simulink library "GenTil_Lib"  (R2023a)
settings: Solver=VariableStepAuto  StartTime=0.0  StopTime=10.0  RelTol=1e-3
values from neighbouring files (symbols this model uses):
  D = [0	0	0	0	0	0	0	0	0	0	0 ... (first row only)    [GenTil.m]
undefined symbols (not defined in the file or in its folder): aircraft, p, phi, psi, q, r, theta, v, w, x, y, z
libraries: simulink_extras x35, simulink x5, matrix_library x4, aerolibatmos2 x1
(part 2 of 2)

== system GenTil_Lib/GenTil/GenTil_Dynamics/Equations_of_Motion_6DoF/Dynamics/Moments/  ==
  note: In mathematics, a skew symmetric matrix is defined as the square matrix that is equal to the negative of its transpose matrix.
      | For any square matrix, A, the transpose matrix is given as A T . A skew-symmetric or antisymmetric matrix A can therefore be represented as, A = -A T .
  X : Inport
  Constant : Constant  Value=0
  Constant1 : Constant  Value=0
  Constant2 : Constant  Value=0
  Demux : Demux  Outputs=3
  From : From
  From1 : From
  Gain3 : Gain  Gain=-1
  Gain4 : Gain  Gain=-1
  Gain5 : Gain  Gain=-1
  Goto : Goto
  Matrix Concatenate3 : Concatenate  NumInputs=3  Mode=Multidimensional array  ConcatenateDimension=2
  Matrix Concatenate4 : Concatenate  NumInputs=3  Mode=Multidimensional array  ConcatenateDimension=2
  Matrix Concatenate5 : Concatenate  NumInputs=3  Mode=Multidimensional array  ConcatenateDimension=2
  Matrix Concatenate6 : Concatenate  NumInputs=3  Mode=Multidimensional array
  skew(x) : Outport
  wires:
  Constant2/1 -> Matrix Concatenate5/3
  Constant1/1 -> Matrix Concatenate4/2
  Constant/1 -> Matrix Concatenate3/1
  Demux/1 -> Goto/1
  Demux/2 -> [B]
  X/1 -> Demux/1
  [B] -> Gain4/1
  From1/1 -> Matrix Concatenate5/2
  Matrix Concatenate3/1 -> Matrix Concatenate6/1
  Demux/3 -> [C]
  [B] -> Matrix Concatenate3/3
  Matrix Concatenate5/1 -> Matrix Concatenate6/3
  Matrix Concatenate6/1 -> skew(x)/1  "skew(x)"
  Gain4/1 -> Matrix Concatenate5/1
  [C] -> Gain5/1
  [C] -> Matrix Concatenate4/1
  Gain3/1 -> Matrix Concatenate4/3
  From/1 -> Gain3/1
  Matrix Concatenate4/1 -> Matrix Concatenate6/2
  Gain5/1 -> Matrix Concatenate3/2

== system GenTil_Lib/GenTil/GenTil_Dynamics/Equations_of_Motion_6DoF/Dynamics/Moments/   ==
  note: In mathematics, a skew symmetric matrix is defined as the square matrix that is equal to the negative of its transpose matrix.
      | For any square matrix, A, the transpose matrix is given as A T . A skew-symmetric or antisymmetric matrix A can therefore be represented as, A = -A T .
  X : Inport
  Constant : Constant  Value=0
  Constant1 : Constant  Value=0
  Constant2 : Constant  Value=0
  Demux : Demux  Outputs=3
  From : From
  From1 : From
  Gain3 : Gain  Gain=-1
  Gain4 : Gain  Gain=-1
  Gain5 : Gain  Gain=-1
  Goto : Goto
  Matrix Concatenate3 : Concatenate  NumInputs=3  Mode=Multidimensional array  ConcatenateDimension=2
  Matrix Concatenate4 : Concatenate  NumInputs=3  Mode=Multidimensional array  ConcatenateDimension=2
  Matrix Concatenate5 : Concatenate  NumInputs=3  Mode=Multidimensional array  ConcatenateDimension=2
  Matrix Concatenate6 : Concatenate  NumInputs=3  Mode=Multidimensional array
  skew(x) : Outport
  wires:
  Constant2/1 -> Matrix Concatenate5/3
  Constant1/1 -> Matrix Concatenate4/2
  Constant/1 -> Matrix Concatenate3/1
  Demux/1 -> Goto/1
  Demux/2 -> [B]
  X/1 -> Demux/1
  [B] -> Gain4/1
  From1/1 -> Matrix Concatenate5/2
  Matrix Concatenate3/1 -> Matrix Concatenate6/1
  Demux/3 -> [C]
  [B] -> Matrix Concatenate3/3
  Matrix Concatenate5/1 -> Matrix Concatenate6/3
  Matrix Concatenate6/1 -> skew(x)/1  "skew(x)"
  Gain4/1 -> Matrix Concatenate5/1
  [C] -> Gain5/1
  [C] -> Matrix Concatenate4/1
  Gain3/1 -> Matrix Concatenate4/3
  From/1 -> Gain3/1
  Matrix Concatenate4/1 -> Matrix Concatenate6/2
  Gain5/1 -> Matrix Concatenate3/2

== system GenTil_Lib/GenTil/GenTil_Dynamics/Equations_of_Motion_6DoF/Dynamics/Moments/      ==
  attitude_angles_rad : Inport
  Product1 : Product  Inputs=3  Multiplication=Matrix(*)
  Subsystem : Subsystem
  C_bv : Outport  PortDimensions=[3,3]
  wires:
  attitude_angles_rad/1 -> Subsystem/1(attitude_angles_rad)
  Product1/1 -> C_bv/1
  Subsystem/3(C_psi) -> Product1/3
  Subsystem/1(C_phi) -> Product1/1
  Subsystem/2(C_theta) -> Product1/2

== system GenTil_Lib/GenTil/GenTil_Dynamics/Equations_of_Motion_6DoF/Dynamics/Moments/ 1 ==
  note: In mathematics, a skew symmetric matrix is defined as the square matrix that is equal to the negative of its transpose matrix.
      | For any square matrix, A, the transpose matrix is given as A T . A skew-symmetric or antisymmetric matrix A can therefore be represented as, A = -A T .
  X : Inport
  Constant : Constant  Value=0
  Constant1 : Constant  Value=0
  Constant2 : Constant  Value=0
  Demux : Demux  Outputs=3
  From : From
  From1 : From
  Gain3 : Gain  Gain=-1
  Gain4 : Gain  Gain=-1
  Gain5 : Gain  Gain=-1
  Goto : Goto
  Matrix Concatenate3 : Concatenate  NumInputs=3  Mode=Multidimensional array  ConcatenateDimension=2
  Matrix Concatenate4 : Concatenate  NumInputs=3  Mode=Multidimensional array  ConcatenateDimension=2
  Matrix Concatenate5 : Concatenate  NumInputs=3  Mode=Multidimensional array  ConcatenateDimension=2
  Matrix Concatenate6 : Concatenate  NumInputs=3  Mode=Multidimensional array
  skew(x) : Outport
  wires:
  Gain5/1 -> Matrix Concatenate3/2
  Matrix Concatenate4/1 -> Matrix Concatenate6/2
  From/1 -> Gain3/1
  Gain3/1 -> Matrix Concatenate4/3
  [C] -> Matrix Concatenate4/1
  [C] -> Gain5/1
  Gain4/1 -> Matrix Concatenate5/1
  Matrix Concatenate6/1 -> skew(x)/1  "skew(x)"
  Matrix Concatenate5/1 -> Matrix Concatenate6/3
  [B] -> Matrix Concatenate3/3
  Demux/3 -> [C]
  Matrix Concatenate3/1 -> Matrix Concatenate6/1
  From1/1 -> Matrix Concatenate5/2
  [B] -> Gain4/1
  X/1 -> Demux/1
  Demux/2 -> [B]
  Demux/1 -> Goto/1
  Constant/1 -> Matrix Concatenate3/1
  Constant1/1 -> Matrix Concatenate4/2
  Constant2/1 -> Matrix Concatenate5/3

== system GenTil_Lib/GenTil/GenTil_Dynamics/Equations_of_Motion_6DoF/Dynamics/Moments/Avoid_Low_Values ==
  In : Inport
  Abs : Abs  SaturateOnIntegerOverflow=off
  Compare To Constant : simulink/Logic and Bit Operations/Compare To Constant  relop=<  const=1e-4  OutDataTypeStr=boolean
  Constant : Constant  Value=0  SampleTime=-1
  Data Type Conversion : DataTypeConversion  OutDataTypeStr=double  SaturateOnIntegerOverflow=off  RndMeth=Floor
  Switch : Switch  Criteria=u2 > Threshold  Threshold=0.05  SaturateOnIntegerOverflow=off  InputSameDT=off
  Out : Outport
  wires:
  Constant/1 -> Switch/1
  Abs/1 -> Compare To Constant/1
  Compare To Constant/1 -> Data Type Conversion/1
  In/1 -> Switch/3, Abs/1
  Data Type Conversion/1 -> Switch/2
  Switch/1 -> Out/1

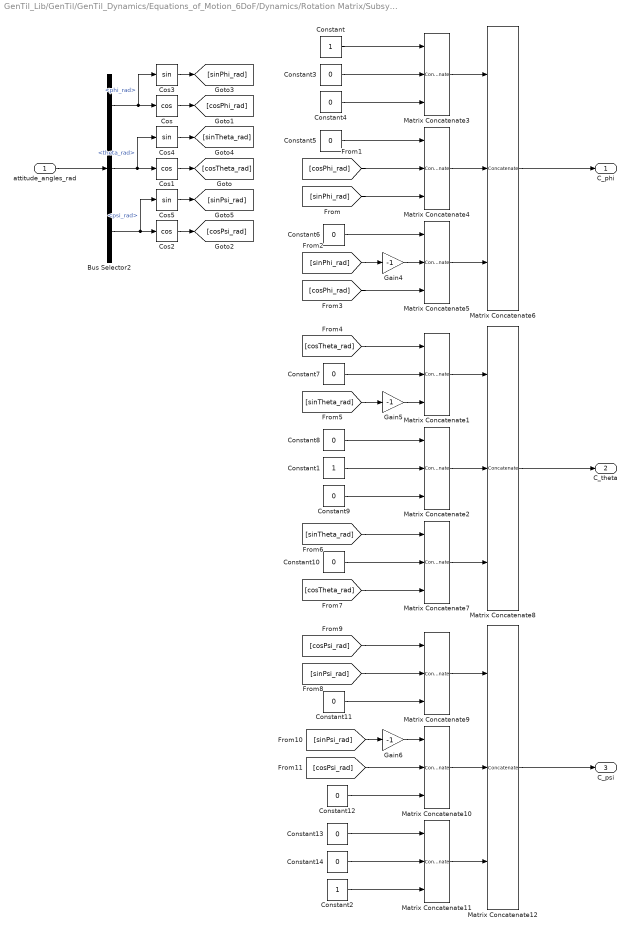
== system GenTil_Lib/GenTil/GenTil_Dynamics/Equations_of_Motion_6DoF/Dynamics/Rotation Matrix/Subsystem ==
  attitude_angles_rad : Inport
  Bus Selector2 : BusSelector  OutputSignals=phi_rad,theta_rad,psi_rad
  Constant : Constant
  Constant1 : Constant
  Constant{3..14} (12 alike) : Constant  Value=0
  Constant2 : Constant
  Cos : Trigonometry  Operator=cos
  Cos1 : Trigonometry  Operator=cos
  Cos2 : Trigonometry  Operator=cos
  Cos3 : Trigonometry
  Cos4 : Trigonometry
  Cos5 : Trigonometry
  Gain4 : Gain  Gain=-1
  Gain5 : Gain  Gain=-1
  Gain6 : Gain  Gain=-1
  Matrix Concatenate{1..5,7,9..11} (9 alike) : Concatenate  NumInputs=3  Mode=Multidimensional array  ConcatenateDimension=2
  Matrix Concatenate12 : Concatenate  NumInputs=3  Mode=Multidimensional array
  Matrix Concatenate6 : Concatenate  NumInputs=3  Mode=Multidimensional array
  Matrix Concatenate8 : Concatenate  NumInputs=3  Mode=Multidimensional array
  C_phi : Outport
  C_theta : Outport  Port=2
  C_psi : Outport  Port=3
  wires:
  Constant14/1 -> Matrix Concatenate11/2
  Constant13/1 -> Matrix Concatenate11/1
  Constant12/1 -> Matrix Concatenate10/3
  Constant11/1 -> Matrix Concatenate9/3
  Constant10/1 -> Matrix Concatenate7/2
  Constant9/1 -> Matrix Concatenate2/3
  Constant8/1 -> Matrix Concatenate2/1
  Constant7/1 -> Matrix Concatenate1/2
  Constant6/1 -> Matrix Concatenate5/1
  Constant5/1 -> Matrix Concatenate4/1
  Constant4/1 -> Matrix Concatenate3/3
  Constant3/1 -> Matrix Concatenate3/2
  [cosPsi_rad] -> Matrix Concatenate10/2
  Matrix Concatenate5/1 -> Matrix Concatenate6/3
  attitude_angles_rad/1 -> Bus Selector2/1
  Matrix Concatenate11/1 -> Matrix Concatenate12/3
  Matrix Concatenate9/1 -> Matrix Concatenate12/1
  [cosTheta_rad] -> Matrix Concatenate7/3
  Matrix Concatenate4/1 -> Matrix Concatenate6/2
  Gain5/1 -> Matrix Concatenate1/3
  [sinPhi_rad] -> Gain4/1
  [cosTheta_rad] -> Matrix Concatenate1/1
  [sinTheta_rad] -> Gain5/1
  Matrix Concatenate7/1 -> Matrix Concatenate8/3
  Matrix Concatenate6/1 -> C_phi/1
  Constant2/1 -> Matrix Concatenate11/3
  Constant/1 -> Matrix Concatenate3/1
  Matrix Concatenate12/1 -> C_psi/1
  Bus Selector2/1 -> Cos/1, Cos3/1  "<phi_rad>"
  Matrix Concatenate3/1 -> Matrix Concatenate6/1
  Cos5/1 -> [sinPsi_rad]
  Matrix Concatenate1/1 -> Matrix Concatenate8/1
  Bus Selector2/3 -> Cos2/1, Cos5/1  "<psi_rad>"
  Cos3/1 -> [sinPhi_rad]
  [cosPhi_rad] -> Matrix Concatenate4/2
  Constant1/1 -> Matrix Concatenate2/2
  Gain6/1 -> Matrix Concatenate10/1
  [cosPhi_rad] -> Matrix Concatenate5/3
  Cos2/1 -> [cosPsi_rad]
  Bus Selector2/2 -> Cos1/1, Cos4/1  "<theta_rad>"
  Matrix Concatenate10/1 -> Matrix Concatenate12/2
  [sinPsi_rad] -> Matrix Concatenate9/2
  Matrix Concatenate8/1 -> C_theta/1
  Cos1/1 -> [cosTheta_rad]
  [sinPhi_rad] -> Matrix Concatenate4/3
  [sinTheta_rad] -> Matrix Concatenate7/1
  Matrix Concatenate2/1 -> Matrix Concatenate8/2
  Gain4/1 -> Matrix Concatenate5/2
  [cosPsi_rad] -> Matrix Concatenate9/1
  [sinPsi_rad] -> Gain6/1
  Cos4/1 -> [sinTheta_rad]
  Cos/1 -> [cosPhi_rad]

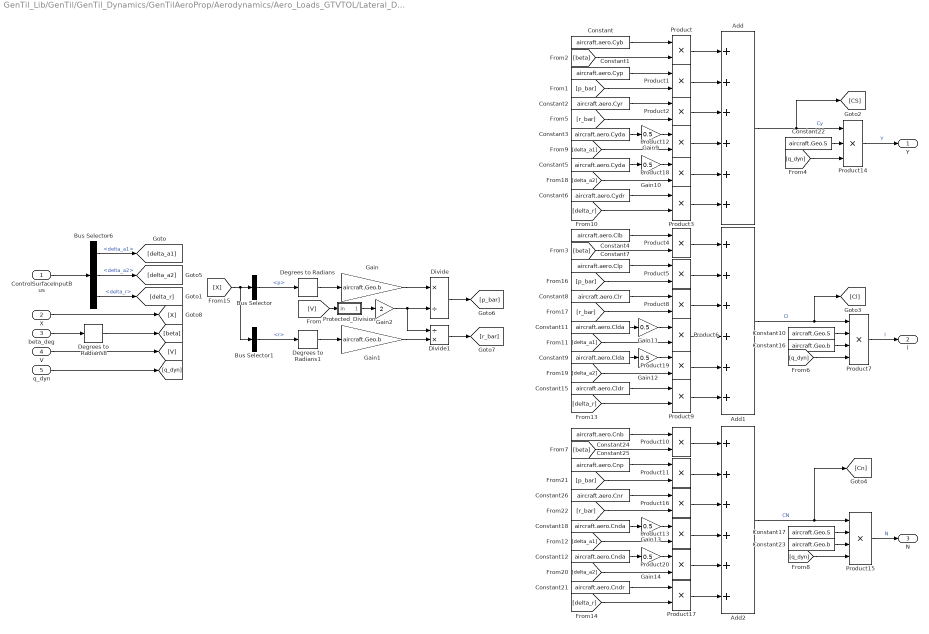
== system GenTil_Lib/GenTil/GenTil_Dynamics/GenTilAeroProp/Aerodynamics/Aero_Loads_GTVTOL/Lateral_Directional_Force_and_Moments ==
  ControlSurfaceInputBus : Inport  OutDataTypeStr=Bus: Actuators
  X : Inport  Port=2  OutDataTypeStr=Bus: States
  beta_deg : Inport  Port=3
  V : Inport  Port=4
  q_dyn : Inport  Port=5
  Add : Sum  Inputs=++++++
  Add1 : Sum  Inputs=++++++
  Add2 : Sum  Inputs=++++++
  Bus Selector : BusSelector  OutputSignals=p
  Bus Selector1 : BusSelector  OutputSignals=r
  Bus Selector6 : BusSelector  OutputSignals=delta_a1,delta_a2,delta_r
  Constant : Constant  Value=aircraft.aero.Cyb
  Constant1 : Constant  Value=aircraft.aero.Cyp
  Constant10 : Constant  Value=aircraft.Geo.S
  Constant11 : Constant  Value=aircraft.aero.Clda
  Constant12 : Constant  Value=aircraft.aero.Cnda
  Constant15 : Constant  Value=aircraft.aero.Cldr
  Constant16 : Constant  Value=aircraft.Geo.b
  Constant17 : Constant  Value=aircraft.Geo.S
  Constant18 : Constant  Value=aircraft.aero.Cnda
  Constant2 : Constant  Value=aircraft.aero.Cyr
  Constant21 : Constant  Value=aircraft.aero.Cndr
  Constant22 : Constant  Value=aircraft.Geo.S
  Constant23 : Constant  Value=aircraft.Geo.b
  Constant24 : Constant  Value=aircraft.aero.Cnb
  Constant25 : Constant  Value=aircraft.aero.Cnp
  Constant26 : Constant  Value=aircraft.aero.Cnr
  Constant3 : Constant  Value=aircraft.aero.Cyda
  Constant4 : Constant  Value=aircraft.aero.Clb
  Constant5 : Constant  Value=aircraft.aero.Cyda
  Constant6 : Constant  Value=aircraft.aero.Cydr
  Constant7 : Constant  Value=aircraft.aero.Clp
  Constant8 : Constant  Value=aircraft.aero.Clr
  Constant9 : Constant  Value=aircraft.aero.Clda
  Degrees to Radians : simulink_extras/Transformations/Degrees to Radians
  Degrees to Radians1 : simulink_extras/Transformations/Degrees to Radians
  Degrees to Radians8 : simulink_extras/Transformations/Degrees to Radians
  Divide : Product  Inputs=*/
  Divide1 : Product  Inputs=/*
  Gain : Gain  Gain=aircraft.Geo.b
  Gain1 : Gain  Gain=aircraft.Geo.b
  Gain{9..14} (6 alike) : Gain  Gain=0.5
  Gain2 : Gain  Gain=2
  Product{,1..6,8..13,16..20} (18 alike) : Product
  Product14 : Product  Inputs=3
  Product15 : Product  Inputs=4
  Product7 : Product  Inputs=4
  Protected_Division : Subsystem
  Y : Outport
  l : Outport  Port=2
  N : Outport  Port=3
  wires:
  Product20/1 -> Add2/5
  Constant12/1 -> Gain14/1
  [delta_a2] -> Product20/2
  Gain14/1 -> Product20/1
  Gain13/1 -> Product13/1
  Product19/1 -> Add1/5
  Constant9/1 -> Gain12/1
  [delta_a2] -> Product19/2
  Gain12/1 -> Product19/1
  Gain11/1 -> Product6/1
  Product18/1 -> Add/5
  [delta_a2] -> Product18/2
  Constant5/1 -> Gain10/1
  Gain10/1 -> Product18/1
  Gain9/1 -> Product12/1
  Bus Selector6/2 -> [delta_a2]  "<delta_a2>"
  Constant4/1 -> Product4/1
  Product14/1 -> Y/1  "Y"
  Gain1/1 -> Divide1/2
  Add1/1 -> [Cl], Product7/1  "Cl"
  Constant21/1 -> Product17/1
  [beta] -> Product10/2
  Bus Selector/1 -> Degrees to Radians/1  "<p>"
  Product5/1 -> Add1/2
  Constant26/1 -> Product16/1
  Divide/1 -> [p_bar]
  [delta_a1] -> Product6/2
  Constant22/1 -> Product14/2
  [delta_r] -> Product17/2
  Constant7/1 -> Product5/1
  Constant17/1 -> Product15/2
  Constant8/1 -> Product8/1
  Constant1/1 -> Product1/1
  Add/1 -> [CS], Product14/1  "Cy"
  Product10/1 -> Add2/1
  Constant3/1 -> Gain9/1
  [delta_a1] -> Product12/2
  Constant10/1 -> Product7/2
  [q_dyn] -> Product15/4
  Product4/1 -> Add1/1
  [q_dyn] -> Product14/3
  [q_dyn] -> Product7/4
  Product7/1 -> l/1  "l"
  Bus Selector1/1 -> Degrees to Radians1/1  "<r>"
  Product13/1 -> Add2/4
  [delta_a1] -> Product13/2
  Product16/1 -> Add2/3
  Product8/1 -> Add1/3
  [beta] -> Product4/2
  Add2/1 -> Product15/1, [Cn]  "CN"
  Constant11/1 -> Gain11/1
  Constant25/1 -> Product11/1
  Constant23/1 -> Product15/3
  Constant6/1 -> Product3/1
  q_dyn/1 -> [q_dyn]
  Constant15/1 -> Product9/1
  V/1 -> [V]
  Gain/1 -> Divide/1
  Constant2/1 -> Product2/1
  Degrees to Radians1/1 -> Gain1/1
  Constant18/1 -> Gain13/1
  Product/1 -> Add/1
  Product12/1 -> Add/4
  Product17/1 -> Add2/6
  [V] -> Protected_Division/1(In)
  Product6/1 -> Add1/4
  Gain2/1 -> Divide1/1, Divide/2
  Constant24/1 -> Product10/1
  Product3/1 -> Add/6
  Degrees to Radians/1 -> Gain/1
  Divide1/1 -> [r_bar]
  Product11/1 -> Add2/2
  Product9/1 -> Add1/6
  Product2/1 -> Add/3
  Constant16/1 -> Product7/3
  Constant/1 -> Product/1
  Product1/1 -> Add/2
  [delta_r] -> Product3/2
  [delta_r] -> Product9/2
  beta_deg/1 -> Degrees to Radians8/1
  Product15/1 -> N/1  "N"
  [beta] -> Product/2
  ControlSurfaceInputBus/1 -> Bus Selector6/1
  Bus Selector6/1 -> [delta_a1]  "<delta_a1>"
  Bus Selector6/3 -> [delta_r]  "<delta_r>"
  Degrees to Radians8/1 -> [beta]
  Protected_Division/1(Out) -> Gain2/1
  X/1 -> [X]
  [X] -> Bus Selector1/1, Bus Selector/1
  [p_bar] -> Product1/2
  [r_bar] -> Product2/2
  [p_bar] -> Product5/2
  [r_bar] -> Product8/2
  [p_bar] -> Product11/2
  [r_bar] -> Product16/2

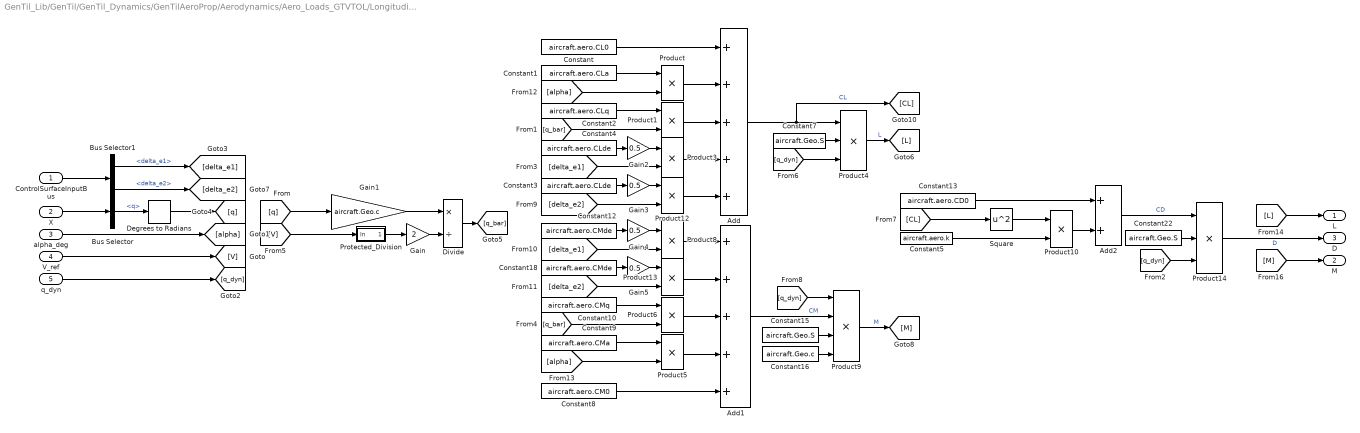
== system GenTil_Lib/GenTil/GenTil_Dynamics/GenTilAeroProp/Aerodynamics/Aero_Loads_GTVTOL/Longitudinal_Forces_and_Moment ==
  ControlSurfaceInputBus : Inport  OutDataTypeStr=Bus: Actuators
  X : Inport  Port=2  OutDataTypeStr=Bus: States
  alpha_deg : Inport  Port=3
  V_ref : Inport  Port=4
  q_dyn : Inport  Port=5
  Add : Sum  Inputs=+++++
  Add1 : Sum  Inputs=+++++
  Add2 : Sum
  Bus Selector : BusSelector  OutputSignals=q
  Bus Selector1 : BusSelector  OutputSignals=delta_e1,delta_e2
  Constant : Constant  Value=aircraft.aero.CL0
  Constant1 : Constant  Value=aircraft.aero.CLa
  Constant10 : Constant  Value=aircraft.aero.CMq
  Constant12 : Constant  Value=aircraft.aero.CMde
  Constant13 : Constant  Value=aircraft.aero.CD0
  Constant15 : Constant  Value=aircraft.Geo.S
  Constant16 : Constant  Value=aircraft.Geo.c
  Constant18 : Constant  Value=aircraft.aero.CMde
  Constant2 : Constant  Value=aircraft.aero.CLq
  Constant22 : Constant  Value=aircraft.Geo.S
  Constant3 : Constant  Value=aircraft.aero.CLde
  Constant4 : Constant  Value=aircraft.aero.CLde
  Constant5 : Constant  Value=aircraft.aero.k
  Constant7 : Constant  Value=aircraft.Geo.S
  Constant8 : Constant  Value=aircraft.aero.CM0
  Constant9 : Constant  Value=aircraft.aero.CMa
  Degrees to Radians : simulink_extras/Transformations/Degrees to Radians
  Divide : Product  Inputs=*/
  Gain : Gain  Gain=2
  Gain1 : Gain  Gain=aircraft.Geo.c
  Gain{2..5} (4 alike) : Gain  Gain=0.5
  Product{,1,3,5..6,8,10,12..13} (9 alike) : Product
  Product14 : Product  Inputs=3
  Product4 : Product  Inputs=3
  Product9 : Product  Inputs=4
  Protected_Division : Subsystem
  Square : Math  Operator=square
  L : Outport
  M : Outport  Port=2
  D : Outport  Port=3
  wires:
  Product13/1 -> Add1/2
  Constant18/1 -> Gain5/1
  Gain5/1 -> Product13/1
  [delta_e2] -> Product13/2
  [delta_e1] -> Product8/2
  Gain4/1 -> Product8/1
  Gain3/1 -> Product12/1
  Gain2/1 -> Product3/1
  [delta_e2] -> Product12/2
  Constant3/1 -> Gain3/1
  [delta_e1] -> Product3/2
  Product12/1 -> Add/5
  Bus Selector1/2 -> [delta_e2]  "<delta_e2>"
  Product/1 -> Add/2
  Constant2/1 -> Product1/1
  Product1/1 -> Add/3
  Add/1 -> [CL], Product4/1  "CL"
  Constant4/1 -> Gain2/1
  Divide/1 -> [q_bar]
  Product4/1 -> [L]  "L"
  q_dyn/1 -> [q_dyn]
  Constant/1 -> Add/1
  Constant7/1 -> Product4/2
  Constant1/1 -> Product/1
  Product3/1 -> Add/4
  Bus Selector/1 -> Degrees to Radians/1  "<q>"
  Constant10/1 -> Product6/1
  Product9/1 -> [M]  "M"
  Constant9/1 -> Product5/1
  Constant12/1 -> Gain4/1
  Constant16/1 -> Product9/4
  Add1/1 -> Product9/2  "CM"
  Constant15/1 -> Product9/3
  Gain/1 -> Divide/2
  X/1 -> Bus Selector/1
  Constant8/1 -> Add1/5
  Product8/1 -> Add1/1
  Product6/1 -> Add1/3
  Degrees to Radians/1 -> [q]
  Constant13/1 -> Add2/1
  Add2/1 -> Product14/1  "CD"
  Constant22/1 -> Product14/2
  Product14/1 -> D/1  "D"
  [q_dyn] -> Product14/3
  Gain1/1 -> Divide/1
  Product5/1 -> Add1/4
  ControlSurfaceInputBus/1 -> Bus Selector1/1
  Bus Selector1/1 -> [delta_e1]  "<delta_e1>"
  Square/1 -> Product10/1
  Constant5/1 -> Product10/2
  Product10/1 -> Add2/2
  Protected_Division/1(Out) -> Gain/1
  V_ref/1 -> [V]
  alpha_deg/1 -> [alpha]
  [q] -> Gain1/1
  [V] -> Protected_Division/1(In)
  [q_dyn] -> Product4/3
  [q_dyn] -> Product9/1
  [alpha] -> Product/2
  [alpha] -> Product5/2
  [q_bar] -> Product1/2
  [q_bar] -> Product6/2
  [CL] -> Square/1
  [L] -> L/1
  [M] -> M/1

== system GenTil_Lib/GenTil/GenTil_Dynamics/GenTilAeroProp/Aerodynamics/Aero_Loads_GTVTOL/Velocity_Check ==
  V_rel : Inport
  rho : Inport  Port=2
  Compare To Constant : simulink/Logic and Bit Operations/Compare To Constant  relop=>=  const=10  OutDataTypeStr=boolean
  Constant : Constant  Value=0  SampleTime=-1
  Data Type Conversion : DataTypeConversion  OutDataTypeStr=double  SaturateOnIntegerOverflow=off  RndMeth=Floor
  Gain : Gain  Gain=0.5
  Product : Product
  Square : Math  Operator=square
  Switch : Switch  Criteria=u2 > Threshold  Threshold=0.05  SaturateOnIntegerOverflow=off  InputSameDT=off
  q_dyn : Outport
  wires:
  Gain/1 -> Product/2
  rho/1 -> Gain/1
  V_rel/1 -> Switch/1, Compare To Constant/1
  Square/1 -> Product/1
  Product/1 -> q_dyn/1
  Compare To Constant/1 -> Data Type Conversion/1
  Data Type Conversion/1 -> Switch/2
  Constant/1 -> Switch/3
  Switch/1 -> Square/1

== system GenTil_Lib/GenTil/GenTil_Dynamics/GenTilAeroProp/Aerodynamics/Aerodynamic_System/Rotation Matrix ==
  attitude_angles_rad : Inport
  Product1 : Product  Inputs=3  Multiplication=Matrix(*)
  Subsystem : Subsystem
  C_bv : Outport  PortDimensions=[3,3]
  wires:
  attitude_angles_rad/1 -> Subsystem/1(attitude_angles_rad)
  Product1/1 -> C_bv/1
  Subsystem/3(C_psi) -> Product1/3
  Subsystem/1(C_phi) -> Product1/1
  Subsystem/2(C_theta) -> Product1/2

== system GenTil_Lib/GenTil/GenTil_Dynamics/GenTilAeroProp/Aerodynamics/Aerodynamic_System/Rotation_Matrix_Alpha_Beta ==
  beta_deg : Inport
  alpha_deg : Inport  Port=2
  Degrees to Radians : simulink_extras/Transformations/Degrees to Radians
  Degrees to Radians1 : simulink_extras/Transformations/Degrees to Radians
  Subsystem : Subsystem
  C_alpha : Outport
  C_beta : Outport  Port=2
  wires:
  Degrees to Radians1/1 -> Subsystem/1(Alpha_rad)
  Degrees to Radians/1 -> Subsystem/2(Beta_rad)
  Subsystem/2(C_beta) -> C_beta/1
  Subsystem/1(C_alpha) -> C_alpha/1
  beta_deg/1 -> Degrees to Radians/1
  alpha_deg/1 -> Degrees to Radians1/1

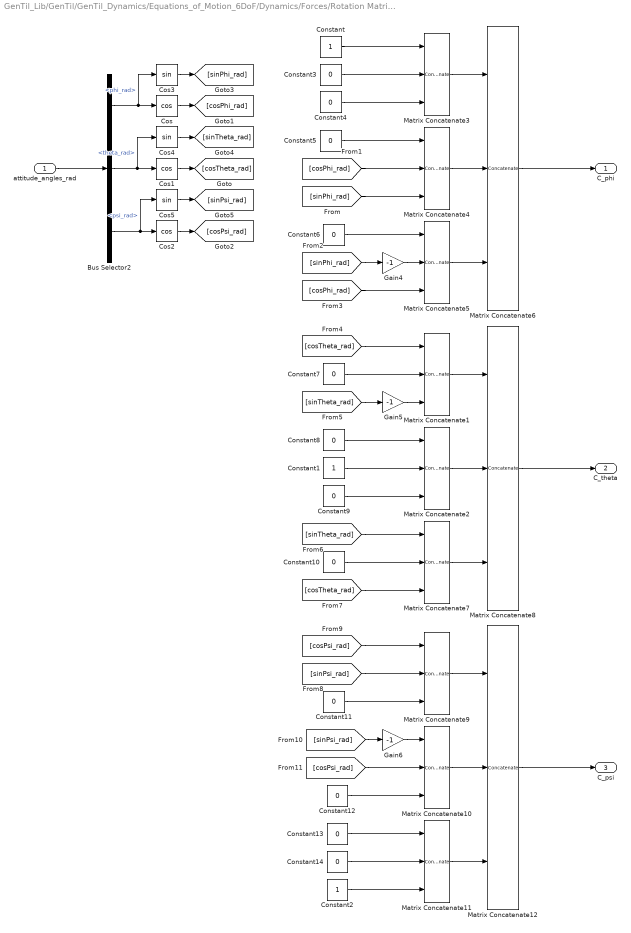
== system GenTil_Lib/GenTil/GenTil_Dynamics/Equations_of_Motion_6DoF/Dynamics/Forces/Rotation Matrix/Subsystem ==
  attitude_angles_rad : Inport
  Bus Selector2 : BusSelector  OutputSignals=phi_rad,theta_rad,psi_rad
  Constant : Constant
  Constant1 : Constant
  Constant{3..14} (12 alike) : Constant  Value=0
  Constant2 : Constant
  Cos : Trigonometry  Operator=cos
  Cos1 : Trigonometry  Operator=cos
  Cos2 : Trigonometry  Operator=cos
  Cos3 : Trigonometry
  Cos4 : Trigonometry
  Cos5 : Trigonometry
  Gain4 : Gain  Gain=-1
  Gain5 : Gain  Gain=-1
  Gain6 : Gain  Gain=-1
  Matrix Concatenate{1..5,7,9..11} (9 alike) : Concatenate  NumInputs=3  Mode=Multidimensional array  ConcatenateDimension=2
  Matrix Concatenate12 : Concatenate  NumInputs=3  Mode=Multidimensional array
  Matrix Concatenate6 : Concatenate  NumInputs=3  Mode=Multidimensional array
  Matrix Concatenate8 : Concatenate  NumInputs=3  Mode=Multidimensional array
  C_phi : Outport
  C_theta : Outport  Port=2
  C_psi : Outport  Port=3
  wires:
  Constant14/1 -> Matrix Concatenate11/2
  Constant13/1 -> Matrix Concatenate11/1
  Constant12/1 -> Matrix Concatenate10/3
  Constant11/1 -> Matrix Concatenate9/3
  Constant10/1 -> Matrix Concatenate7/2
  Constant9/1 -> Matrix Concatenate2/3
  Constant8/1 -> Matrix Concatenate2/1
  Constant7/1 -> Matrix Concatenate1/2
  Constant6/1 -> Matrix Concatenate5/1
  Constant5/1 -> Matrix Concatenate4/1
  Constant4/1 -> Matrix Concatenate3/3
  Constant3/1 -> Matrix Concatenate3/2
  [cosPsi_rad] -> Matrix Concatenate10/2
  Matrix Concatenate5/1 -> Matrix Concatenate6/3
  attitude_angles_rad/1 -> Bus Selector2/1
  Matrix Concatenate11/1 -> Matrix Concatenate12/3
  Matrix Concatenate9/1 -> Matrix Concatenate12/1
  [cosTheta_rad] -> Matrix Concatenate7/3
  Matrix Concatenate4/1 -> Matrix Concatenate6/2
  Gain5/1 -> Matrix Concatenate1/3
  [sinPhi_rad] -> Gain4/1
  [cosTheta_rad] -> Matrix Concatenate1/1
  [sinTheta_rad] -> Gain5/1
  Matrix Concatenate7/1 -> Matrix Concatenate8/3
  Matrix Concatenate6/1 -> C_phi/1
  Constant2/1 -> Matrix Concatenate11/3
  Constant/1 -> Matrix Concatenate3/1
  Matrix Concatenate12/1 -> C_psi/1
  Bus Selector2/1 -> Cos/1, Cos3/1  "<phi_rad>"
  Matrix Concatenate3/1 -> Matrix Concatenate6/1
  Cos5/1 -> [sinPsi_rad]
  Matrix Concatenate1/1 -> Matrix Concatenate8/1
  Bus Selector2/3 -> Cos2/1, Cos5/1  "<psi_rad>"
  Cos3/1 -> [sinPhi_rad]
  [cosPhi_rad] -> Matrix Concatenate4/2
  Constant1/1 -> Matrix Concatenate2/2
  Gain6/1 -> Matrix Concatenate10/1
  [cosPhi_rad] -> Matrix Concatenate5/3
  Cos2/1 -> [cosPsi_rad]
  Bus Selector2/2 -> Cos1/1, Cos4/1  "<theta_rad>"
  Matrix Concatenate10/1 -> Matrix Concatenate12/2
  [sinPsi_rad] -> Matrix Concatenate9/2
  Matrix Concatenate8/1 -> C_theta/1
  Cos1/1 -> [cosTheta_rad]
  [sinPhi_rad] -> Matrix Concatenate4/3
  [sinTheta_rad] -> Matrix Concatenate7/1
  Matrix Concatenate2/1 -> Matrix Concatenate8/2
  Gain4/1 -> Matrix Concatenate5/2
  [cosPsi_rad] -> Matrix Concatenate9/1
  [sinPsi_rad] -> Gain6/1
  Cos4/1 -> [sinTheta_rad]
  Cos/1 -> [cosPhi_rad]

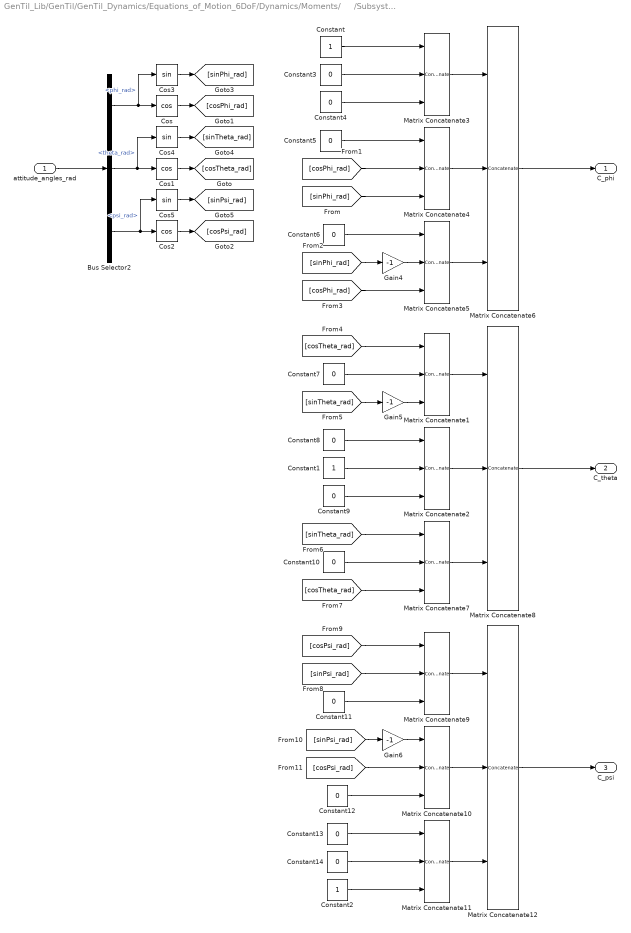
== system GenTil_Lib/GenTil/GenTil_Dynamics/Equations_of_Motion_6DoF/Dynamics/Moments/     /Subsystem ==
  attitude_angles_rad : Inport
  Bus Selector2 : BusSelector  OutputSignals=phi_rad,theta_rad,psi_rad
  Constant : Constant
  Constant1 : Constant
  Constant{3..14} (12 alike) : Constant  Value=0
  Constant2 : Constant
  Cos : Trigonometry  Operator=cos
  Cos1 : Trigonometry  Operator=cos
  Cos2 : Trigonometry  Operator=cos
  Cos3 : Trigonometry
  Cos4 : Trigonometry
  Cos5 : Trigonometry
  Gain4 : Gain  Gain=-1
  Gain5 : Gain  Gain=-1
  Gain6 : Gain  Gain=-1
  Matrix Concatenate{1..5,7,9..11} (9 alike) : Concatenate  NumInputs=3  Mode=Multidimensional array  ConcatenateDimension=2
  Matrix Concatenate12 : Concatenate  NumInputs=3  Mode=Multidimensional array
  Matrix Concatenate6 : Concatenate  NumInputs=3  Mode=Multidimensional array
  Matrix Concatenate8 : Concatenate  NumInputs=3  Mode=Multidimensional array
  C_phi : Outport
  C_theta : Outport  Port=2
  C_psi : Outport  Port=3
  wires:
  Constant14/1 -> Matrix Concatenate11/2
  Constant13/1 -> Matrix Concatenate11/1
  Constant12/1 -> Matrix Concatenate10/3
  Constant11/1 -> Matrix Concatenate9/3
  Constant10/1 -> Matrix Concatenate7/2
  Constant9/1 -> Matrix Concatenate2/3
  Constant8/1 -> Matrix Concatenate2/1
  Constant7/1 -> Matrix Concatenate1/2
  Constant6/1 -> Matrix Concatenate5/1
  Constant5/1 -> Matrix Concatenate4/1
  Constant4/1 -> Matrix Concatenate3/3
  Constant3/1 -> Matrix Concatenate3/2
  [cosPsi_rad] -> Matrix Concatenate10/2
  Matrix Concatenate5/1 -> Matrix Concatenate6/3
  attitude_angles_rad/1 -> Bus Selector2/1
  Matrix Concatenate11/1 -> Matrix Concatenate12/3
  Matrix Concatenate9/1 -> Matrix Concatenate12/1
  [cosTheta_rad] -> Matrix Concatenate7/3
  Matrix Concatenate4/1 -> Matrix Concatenate6/2
  Gain5/1 -> Matrix Concatenate1/3
  [sinPhi_rad] -> Gain4/1
  [cosTheta_rad] -> Matrix Concatenate1/1
  [sinTheta_rad] -> Gain5/1
  Matrix Concatenate7/1 -> Matrix Concatenate8/3
  Matrix Concatenate6/1 -> C_phi/1
  Constant2/1 -> Matrix Concatenate11/3
  Constant/1 -> Matrix Concatenate3/1
  Matrix Concatenate12/1 -> C_psi/1
  Bus Selector2/1 -> Cos/1, Cos3/1  "<phi_rad>"
  Matrix Concatenate3/1 -> Matrix Concatenate6/1
  Cos5/1 -> [sinPsi_rad]
  Matrix Concatenate1/1 -> Matrix Concatenate8/1
  Bus Selector2/3 -> Cos2/1, Cos5/1  "<psi_rad>"
  Cos3/1 -> [sinPhi_rad]
  [cosPhi_rad] -> Matrix Concatenate4/2
  Constant1/1 -> Matrix Concatenate2/2
  Gain6/1 -> Matrix Concatenate10/1
  [cosPhi_rad] -> Matrix Concatenate5/3
  Cos2/1 -> [cosPsi_rad]
  Bus Selector2/2 -> Cos1/1, Cos4/1  "<theta_rad>"
  Matrix Concatenate10/1 -> Matrix Concatenate12/2
  [sinPsi_rad] -> Matrix Concatenate9/2
  Matrix Concatenate8/1 -> C_theta/1
  Cos1/1 -> [cosTheta_rad]
  [sinPhi_rad] -> Matrix Concatenate4/3
  [sinTheta_rad] -> Matrix Concatenate7/1
  Matrix Concatenate2/1 -> Matrix Concatenate8/2
  Gain4/1 -> Matrix Concatenate5/2
  [cosPsi_rad] -> Matrix Concatenate9/1
  [sinPsi_rad] -> Gain6/1
  Cos4/1 -> [sinTheta_rad]
  Cos/1 -> [cosPhi_rad]

== system GenTil_Lib/GenTil/GenTil_Dynamics/GenTilAeroProp/Aerodynamics/Aero_Loads_GTVTOL/Lateral_Directional_Force_and_Moments/Protected_Division ==
  In : Inport
  Add1 : Sum
  Constant : Constant  Value=1e-6
  Out : Outport
  wires:
  In/1 -> Add1/1
  Constant/1 -> Add1/2
  Add1/1 -> Out/1

== system GenTil_Lib/GenTil/GenTil_Dynamics/GenTilAeroProp/Aerodynamics/Aero_Loads_GTVTOL/Longitudinal_Forces_and_Moment/Protected_Division ==
  In : Inport
  Add1 : Sum
  Constant : Constant  Value=1e-6
  Out : Outport
  wires:
  In/1 -> Add1/1
  Constant/1 -> Add1/2
  Add1/1 -> Out/1

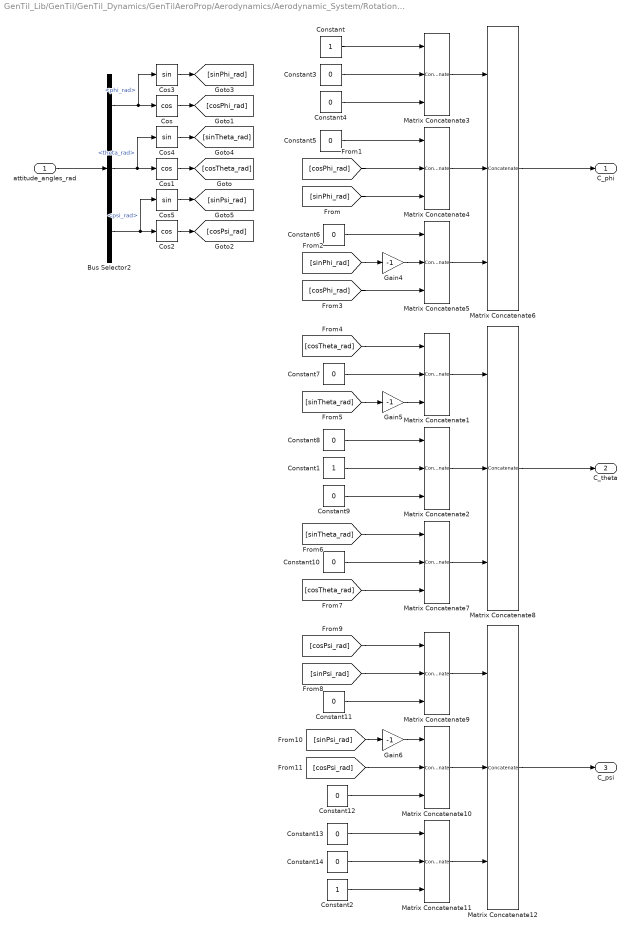
== system GenTil_Lib/GenTil/GenTil_Dynamics/GenTilAeroProp/Aerodynamics/Aerodynamic_System/Rotation Matrix/Subsystem ==
  attitude_angles_rad : Inport
  Bus Selector2 : BusSelector  OutputSignals=phi_rad,theta_rad,psi_rad
  Constant : Constant
  Constant1 : Constant
  Constant{3..14} (12 alike) : Constant  Value=0
  Constant2 : Constant
  Cos : Trigonometry  Operator=cos
  Cos1 : Trigonometry  Operator=cos
  Cos2 : Trigonometry  Operator=cos
  Cos3 : Trigonometry
  Cos4 : Trigonometry
  Cos5 : Trigonometry
  Gain4 : Gain  Gain=-1
  Gain5 : Gain  Gain=-1
  Gain6 : Gain  Gain=-1
  Matrix Concatenate{1..5,7,9..11} (9 alike) : Concatenate  NumInputs=3  Mode=Multidimensional array  ConcatenateDimension=2
  Matrix Concatenate12 : Concatenate  NumInputs=3  Mode=Multidimensional array
  Matrix Concatenate6 : Concatenate  NumInputs=3  Mode=Multidimensional array
  Matrix Concatenate8 : Concatenate  NumInputs=3  Mode=Multidimensional array
  C_phi : Outport
  C_theta : Outport  Port=2
  C_psi : Outport  Port=3
  wires:
  Constant14/1 -> Matrix Concatenate11/2
  Constant13/1 -> Matrix Concatenate11/1
  Constant12/1 -> Matrix Concatenate10/3
  Constant11/1 -> Matrix Concatenate9/3
  Constant10/1 -> Matrix Concatenate7/2
  Constant9/1 -> Matrix Concatenate2/3
  Constant8/1 -> Matrix Concatenate2/1
  Constant7/1 -> Matrix Concatenate1/2
  Constant6/1 -> Matrix Concatenate5/1
  Constant5/1 -> Matrix Concatenate4/1
  Constant4/1 -> Matrix Concatenate3/3
  Constant3/1 -> Matrix Concatenate3/2
  [cosPsi_rad] -> Matrix Concatenate10/2
  Matrix Concatenate5/1 -> Matrix Concatenate6/3
  attitude_angles_rad/1 -> Bus Selector2/1
  Matrix Concatenate11/1 -> Matrix Concatenate12/3
  Matrix Concatenate9/1 -> Matrix Concatenate12/1
  [cosTheta_rad] -> Matrix Concatenate7/3
  Matrix Concatenate4/1 -> Matrix Concatenate6/2
  Gain5/1 -> Matrix Concatenate1/3
  [sinPhi_rad] -> Gain4/1
  [cosTheta_rad] -> Matrix Concatenate1/1
  [sinTheta_rad] -> Gain5/1
  Matrix Concatenate7/1 -> Matrix Concatenate8/3
  Matrix Concatenate6/1 -> C_phi/1
  Constant2/1 -> Matrix Concatenate11/3
  Constant/1 -> Matrix Concatenate3/1
  Matrix Concatenate12/1 -> C_psi/1
  Bus Selector2/1 -> Cos/1, Cos3/1  "<phi_rad>"
  Matrix Concatenate3/1 -> Matrix Concatenate6/1
  Cos5/1 -> [sinPsi_rad]
  Matrix Concatenate1/1 -> Matrix Concatenate8/1
  Bus Selector2/3 -> Cos2/1, Cos5/1  "<psi_rad>"
  Cos3/1 -> [sinPhi_rad]
  [cosPhi_rad] -> Matrix Concatenate4/2
  Constant1/1 -> Matrix Concatenate2/2
  Gain6/1 -> Matrix Concatenate10/1
  [cosPhi_rad] -> Matrix Concatenate5/3
  Cos2/1 -> [cosPsi_rad]
  Bus Selector2/2 -> Cos1/1, Cos4/1  "<theta_rad>"
  Matrix Concatenate10/1 -> Matrix Concatenate12/2
  [sinPsi_rad] -> Matrix Concatenate9/2
  Matrix Concatenate8/1 -> C_theta/1
  Cos1/1 -> [cosTheta_rad]
  [sinPhi_rad] -> Matrix Concatenate4/3
  [sinTheta_rad] -> Matrix Concatenate7/1
  Matrix Concatenate2/1 -> Matrix Concatenate8/2
  Gain4/1 -> Matrix Concatenate5/2
  [cosPsi_rad] -> Matrix Concatenate9/1
  [sinPsi_rad] -> Gain6/1
  Cos4/1 -> [sinTheta_rad]
  Cos/1 -> [cosPhi_rad]

== system GenTil_Lib/GenTil/GenTil_Dynamics/GenTilAeroProp/Aerodynamics/Aerodynamic_System/Rotation_Matrix_Alpha_Beta/Subsystem ==
  Alpha_rad : Inport
  Beta_rad : Inport  Port=2
  Constant{,3..9} (8 alike) : Constant  Value=0
  Constant1 : Constant
  Constant2 : Constant
  Cos1 : Trigonometry  Operator=cos
  Cos2 : Trigonometry  Operator=cos
  Cos4 : Trigonometry
  Cos5 : Trigonometry
  Gain5 : Gain  Gain=-1
  Gain6 : Gain  Gain=-1
  Matrix Concatenate{1..2,7,9..11} (6 alike) : Concatenate  NumInputs=3  Mode=Multidimensional array  ConcatenateDimension=2
  Matrix Concatenate12 : Concatenate  NumInputs=3  Mode=Multidimensional array
  Matrix Concatenate8 : Concatenate  NumInputs=3  Mode=Multidimensional array
  C_alpha : Outport
  C_beta : Outport  Port=2
  wires:
  Constant9/1 -> Matrix Concatenate1/2
  Constant8/1 -> Matrix Concatenate11/2
  Constant7/1 -> Matrix Concatenate11/1
  Constant6/1 -> Matrix Concatenate10/3
  Constant5/1 -> Matrix Concatenate9/3
  Constant4/1 -> Matrix Concatenate7/2
  Constant3/1 -> Matrix Concatenate2/3
  Constant/1 -> Matrix Concatenate2/1
  [cosBeta_rad] -> Matrix Concatenate10/2
  Matrix Concatenate11/1 -> Matrix Concatenate12/3
  Matrix Concatenate9/1 -> Matrix Concatenate12/1
  [cosAlpha_rad] -> Matrix Concatenate7/3
  Gain5/1 -> Matrix Concatenate1/3
  [cosAlpha_rad] -> Matrix Concatenate1/1
  [sinAlpha_rad] -> Gain5/1
  Matrix Concatenate7/1 -> Matrix Concatenate8/3
  Constant2/1 -> Matrix Concatenate11/3
  Matrix Concatenate12/1 -> C_beta/1
  Cos5/1 -> [sinBeta_rad]
  Matrix Concatenate1/1 -> Matrix Concatenate8/1
  Beta_rad/1 -> Cos2/1, Cos5/1
  Constant1/1 -> Matrix Concatenate2/2
  Gain6/1 -> Matrix Concatenate10/1
  Cos2/1 -> [cosBeta_rad]
  Alpha_rad/1 -> Cos1/1, Cos4/1
  Matrix Concatenate10/1 -> Matrix Concatenate12/2
  [sinBeta_rad] -> Matrix Concatenate9/2
  Matrix Concatenate8/1 -> C_alpha/1
  Cos1/1 -> [cosAlpha_rad]
  [sinAlpha_rad] -> Matrix Concatenate7/1
  Matrix Concatenate2/1 -> Matrix Concatenate8/2
  [cosBeta_rad] -> Matrix Concatenate9/1
  [sinBeta_rad] -> Gain6/1
  Cos4/1 -> [sinAlpha_rad]
